simulink model "ident2"  (Simulink 4.00)
settings: Solver=ode45  StartTime=0.0  StopTime=30  MaxStep=0.1  RelTol=1e-3
values from neighbouring files (symbols this model uses):
  k = 0.998681225655    [ident21.mat]    (also in ncd_kalm_1.mat = [20.04 41.6748 91.25676 100.22352 54.94452 22.0392]; ncd_kalm_2.mat = [20.04 41.6748 91.25676 100.22352 54.94452 22.0392]; ncd_pol1.m = place(A, B, p); ncd_pol_1.mat = [20.04 41.6748 91.25676 100.22352 54.94452 22.0392])
  tau = 1.00031317223    [ident21.mat]
  zetha = 0.0500614532492    [ident21.mat]
settings Model: LastModifiedBy=Administrator  BlockReductionOpt=off

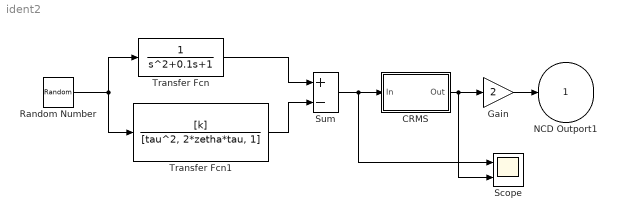
== system ident2 ==
  CRMS : Subsystem
      settings: RTWFcnNameOpts=Auto  RTWFileNameOpts=Auto
      mask Type: Continuous RMS Value Block
      mask Description: Computes the cumulative root mean squared value of the input signal. The output is continuous.
      mask Display: disp('Continuous\nRMS');
  Gain : Gain  Gain=2  Multiplication=Element-wise(K.*u)  SaturateOnIntegerOverflow=on
  Random Number : RandomNumber  Mean=0  Variance=1  Seed=0  SampleTime=0
  Scope : Scope  NumInputPorts=2
      settings: TimeRange=auto  YMin=-1~1.16495  YMax=1~1.16495  SaveToWorkspace=off  SaveName=ScopeData  LimitDataPoints=on  MaxDataPoints=5000
  Sum : Sum  Inputs=+-  SaturateOnIntegerOverflow=on
  Transfer Fcn : TransferFcn  Numerator=[1]  Denominator=[1 0.1 1]  Realization=auto  AbsoluteTolerance=auto
  Transfer Fcn1 : TransferFcn  Numerator=[k]  Denominator=[tau^2, 2*zetha*tau, 1]  Realization=auto  AbsoluteTolerance=auto
  NCD Outport1 : Outport  Port=1  InitialOutput=0
      settings: OpenFcn=optblock
      mask Type: NCD Outport
      mask Display:
      | plot([0:10],[-.5 1.5 .6 1.3 .8 1.1 .95 1.02 .99 1 1]);
      | disp('\n\n NCD\n OutPort 1');
  wires:
  Random Number/1 -> Transfer Fcn1/1, Transfer Fcn/1
  Transfer Fcn/1 -> Sum/1
  Transfer Fcn1/1 -> Sum/2
  Sum/1 -> CRMS/1(In), Scope/1
  CRMS/1(Out) -> Scope/2, Gain/1
  Gain/1 -> NCD Outport1/1

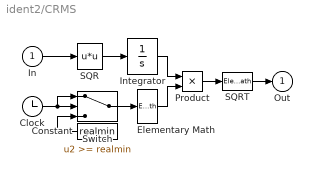
== system ident2/CRMS ==
  In : Inport  Port=1
  Clock : Clock
      settings: DisplayTime=off  Decimation=10
  Constant : Constant  Orientation=left  Value=realmin
  Elementary Math : ElementaryMath  Operator=reciprocal
  Integrator : Integrator  ExternalReset=none  InitialConditionSource=internal  InitialCondition=0  LimitOutput=on  UpperSaturationLimit=inf  LowerSaturationLimit=0  ShowSaturationPort=off  ShowStatePort=off  AbsoluteTolerance=auto
  Product : Product  Inputs=2  Multiplication=Element-wise(.*)  SaturateOnIntegerOverflow=on
  SQR : Fcn  Expr=u*u
  SQRT : ElementaryMath  Operator=sqrt
  Switch : Switch  Threshold=realmin
  Out : Outport  Port=1  InitialOutput=0
  wires:
  In/1 -> SQR/1
  SQR/1 -> Integrator/1
  Integrator/1 -> Product/1
  Switch/1 -> Elementary Math/1
  Clock/1 -> Switch/2, Switch/1
  Constant/1 -> Switch/3
  Elementary Math/1 -> Product/2
  SQRT/1 -> Out/1
  Product/1 -> SQRT/1
